simulink model "clase07simulink"  (R2019b)
settings: Solver=VariableStepAuto  StartTime=0.0  StopTime=10.0  RelTol=1e-3
undefined symbols (not defined in the file): A, B, C, D, xini
settings Model: Creator=B13  LastModifiedBy=B13

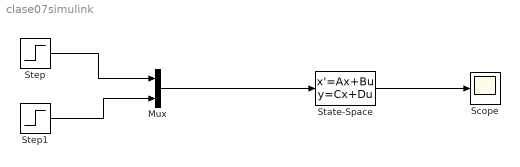
== system clase07simulink ==
  Mux : Mux  Inputs=2
  Scope : Scope
  State-Space : StateSpace  A=A  B=B  C=C  D=D  InitialCondition=xini
  Step : Step  Time=0  SampleTime=0
  Step1 : Step  Time=0  After=0.2  SampleTime=0
  wires:
  Mux/1 -> State-Space/1
  Step/1 -> Mux/1
  Step1/1 -> Mux/2
  State-Space/1 -> Scope/1
